simulink model "H_infinitude"  (R2020a)
settings: Solver=VariableStepAuto  StartTime=0.0  StopTime=10.0  RelTol=1e-3
values from neighbouring files (symbols this model uses):
  A = [0,0,1,0 ;0,0,0,1 ;k1,0,0,0 ;k2,0,0,0]    [Parameters.m]
  B1 = [0;0;0.2;0.2]    [Parameters.m]
  B2 = [0; 0; k3; k4]    [Parameters.m]
  K = W/X    [LMIC.m]    (also in Parameters.m = LMIC(A,B1,B2,C1,D11,D12,gamma,N))
  x0 = [1,2,2,1]/2    [Parameters.m]
settings Model: Creator=18423  LastModifiedBy=18423

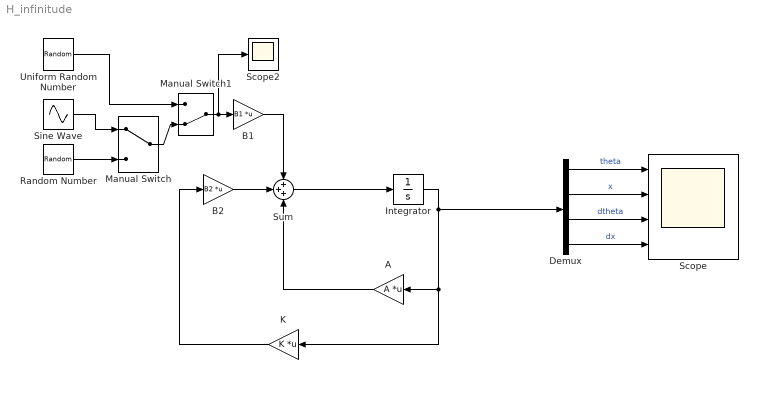
== system H_infinitude ==
  A : Gain  Gain=A  Multiplication=Matrix(K*u)
  B1 : Gain  Gain=B1  Multiplication=Matrix(K*u)
  B2 : Gain  Gain=B2  Multiplication=Matrix(K*u)
  Demux : Demux
  Integrator : Integrator  InitialCondition=x0
  K : Gain  Gain=K  Multiplication=Matrix(K*u)
  Manual Switch : ManualSwitch
  Manual Switch1 : ManualSwitch  CurrentSetting=0
  Random Number : RandomNumber  SampleTime=0.0001
  Scope : Scope  NumInputPorts=4
  Scope2 : Scope
  Sine Wave : Sin  Amplitude=2  Frequency=200  SampleTime=0
  Sum : Sum  Inputs=+++
  Uniform Random Number : UniformRandomNumber  Minimum=-2  Maximum=2  SampleTime=0.001
  wires:
  Sum/1 -> Integrator/1
  Integrator/1 -> K/1, A/1, Demux/1
  A/1 -> Sum/3
  Demux/1 -> Scope/1  "theta"
  Demux/2 -> Scope/2  "x"
  Demux/3 -> Scope/3  "dtheta"
  Demux/4 -> Scope/4  "dx"
  B1/1 -> Sum/1
  B2/1 -> Sum/2
  K/1 -> B2/1
  Random Number/1 -> Manual Switch/2
  Sine Wave/1 -> Manual Switch/1
  Manual Switch/1 -> Manual Switch1/2
  Uniform Random Number/1 -> Manual Switch1/1
  Manual Switch1/1 -> Scope2/1, B1/1
